simulink model "quatercar_simulinkmodel"  (R2025a)
settings: Solver=VariableStepAuto  StartTime=0.0  StopTime=10  RelTol=1e-3
values from neighbouring files (symbols this model uses):
  b = 300    [param_quatercarmodel.m]
  c = 10000    [param_quatercarmodel.m]
  c_us = 1000    [param_quatercarmodel.m]
  G = 10000    [param_quatercarmodel.m]
  m = 300    [param_quatercarmodel.m]
  m_us = 40    [param_quatercarmodel.m]
libraries: slpidlib x2
settings Model: Creator=TARUN NAIDU  LastModifiedBy=TARUN NAIDU

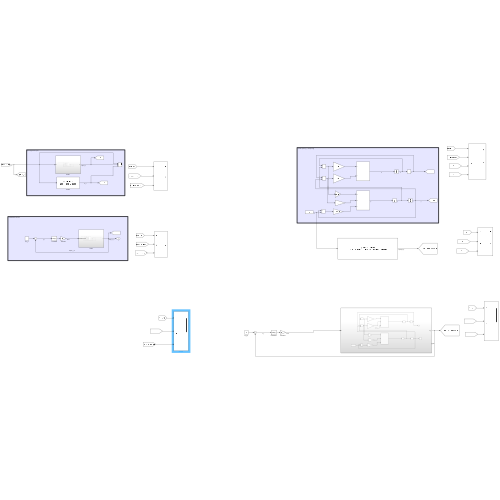
[thumbnail: Simulink's stored preview of the top-level diagram]
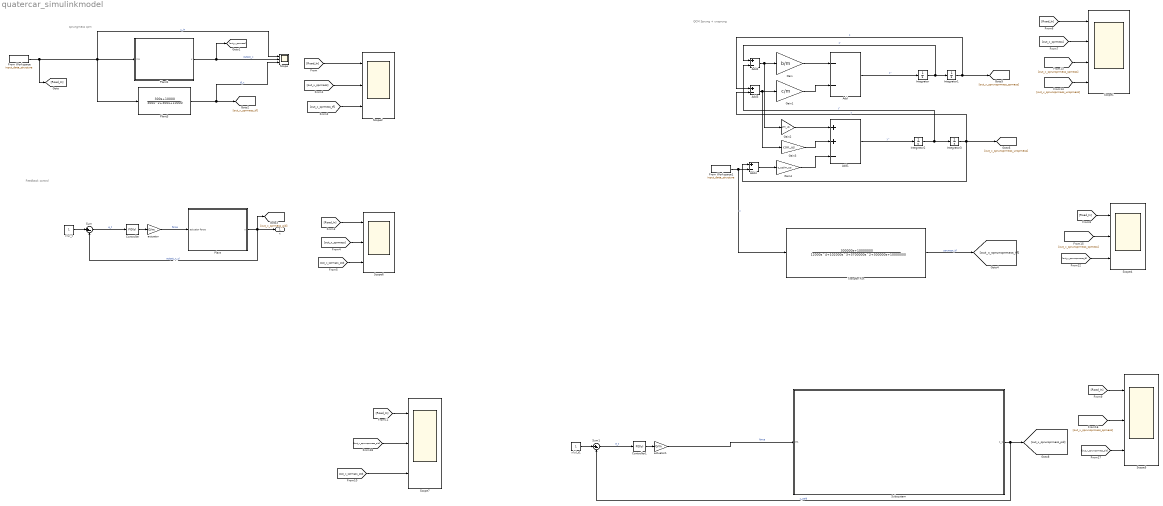
== system quatercar_simulinkmodel ==
  note: sprungmass qcm
  note: Feedback control
  note: QCM Sprung + unsprung
  Add : Sum  Inputs=--
  Add1 : Sum  Inputs=++-
  Add2 : Sum  Inputs=+-
  Add3 : Sum  Inputs=+-
  Add4 : Sum  Inputs=+-
  Controller : slpidlib/PID Controller  Controller=PID  Form=Parallel  TimeDomain=Continuous-time  UseExternalTs=off  SampleTime=-1  IntegratorMethod=Forward Euler  FilterMethod=Forward Euler  ControllerParametersSource=internal  P=4.4259  I=11.6475  UseKiTs=off  D=0.37311  UseExternalDerivativeSource=off  N=100  UseFilter=on  TunerSelectOption=Transfer Function Based (PID Tuner App)  InitialConditionSource=internal  InitialConditionForIntegrator=0  InitialConditionForFilter=0  DifferentiatorICPrevScaledInput=0  ExternalReset=none  TrackingMode=off  Kt=1  LimitOutput=off  SatLimitsSource=internal  UpperSaturationLimit=inf  LowerSaturationLimit=-inf  LinearizeAsGain=on  AntiWindupMode=none  Kb=1  LimitIntegrator=off  UpperIntegratorSaturationLimit=inf  LowerIntegratorSaturationLimit=-inf  POutMin=[]  POutMax=[]  IOutMin=[]  IOutMax=[]  DOutMin=[]  DOutMax=[]  NOutMin=[]  NOutMax=[]  SumOutMin=[]  SumOutMax=[]  SaturationOutMin=[]  SaturationOutMax=[]  PParamMin=[]  PParamMax=[]  IParamMin=[]  IParamMax=[]  DParamMin=[]  DParamMax=[]  NParamMin=[]  NParamMax=[]  KbParamMin=[]  KbParamMax=[]  KtParamMin=[]  KtParamMax=[]  KbOutMin=[]  KbOutMax=[]  KtOutMin=[]  KtOutMax=[]  IntegratorOutMin=[]  IntegratorOutMax=[]  FilterOutMin=[]  FilterOutMax=[]  SumI1OutMin=[]  SumI1OutMax=[]  SumI2OutMin=[]  SumI2OutMax=[]  SumI3OutMin=[]  SumI3OutMax=[]  SumI4OutMin=[]  SumI4OutMax=[]  SumDOutMin=[]  SumDOutMax=[]  DifferentiatorOutMin=[]  DifferentiatorOutMax=[]  FilterDiffOutCoefMin=[]  FilterDiffOutCoefMax=[]  ReciprocalOutMin=[]  ReciprocalOutMax=[]  SumDenOutMin=[]  SumDenOutMax=[]  SumNumOutMin=[]  SumNumOutMax=[]  DivideOutMin=[]  DivideOutMax=[]  UdiffTsProdOutMin=[]  UdiffTsProdOutMax=[]  NTsProdOutMin=[]  NTsProdOutMax=[]  UintegralTsProdOutMin=[]  UintegralTsProdOutMax=[]  UngainTsProdOutMin=[]  UngainTsProdOutMax=[]  ClampingZeroOutDataTypeStr=Inherit: Inherit via back propagation  ClampingZeroOutMin=[]  ClampingZeroOutMax=[]  FilterDenConstantOutDataTypeStr=Inherit: Inherit via back propagation  FilterDenConstantOutMin=[]  FilterDenConstantOutMax=[]  PCopyOutDataTypeStr=Inherit: Inherit via back propagation  PCopyOutMin=[]  PCopyOutMax=[]  NCopyOutDataTypeStr=Inherit: Inherit via back propagation  NCopyOutMin=[]  NCopyOutMax=[]  IntegratorContinuousStateAttributes=''  IntegratorStateMustResolveToSignalObject=off  IntegratorRTWStateStorageClass=Auto  FilterContinuousStateAttributes=''  FilterStateMustResolveToSignalObject=off  FilterRTWStateStorageClass=Auto  ParallelPVariant=InternalParameters  IdealPVariant=Disabled  IVariant=InternalParameters  DVariant=InternalParameters  IntegratorVariant=Continuous  SatVariant=Disabled  AWVariant=Passthrough  PCopyVariant=Disabled  TRVariant=Disabled  FdbkBlocksVariant=Forward  IdealPFdbkVariant=Disabled  SatFdbkVariant=Disabled  DerivativeFilterVariant=ContFilter  NVariant=InternalParameters  NCopyVariant=Disabled  FilterICVariant=InternalICsFilter  IntegratorICVariant=InternalICs  ExternalResetVariant=Disabled  TRSumVariant=Passthrough  SumFdbkVariant=Disabled  SumVariant=Sum_PID  TsampFilterVariant=InternalTs  TsampNgainVariant=Passthrough  TsampIntegralVariant=Disabled_SignalSpec  ExternalSaturationOutDataTypeStr=Inherit: Same as second input  DerivativeSourceVariant=ErrorSignal  PreIntVariant=InternalPreInt
  Controller1 : slpidlib/PID Controller  Controller=PID  Form=Parallel  TimeDomain=Continuous-time  UseExternalTs=off  SampleTime=-1  IntegratorMethod=Forward Euler  FilterMethod=Forward Euler  ControllerParametersSource=internal  P=4.8162  I=3.2747  UseKiTs=off  D=1.5851  UseExternalDerivativeSource=off  N=100  UseFilter=on  TunerSelectOption=Transfer Function Based (PID Tuner App)  InitialConditionSource=internal  InitialConditionForIntegrator=0  InitialConditionForFilter=0  DifferentiatorICPrevScaledInput=0  ExternalReset=none  TrackingMode=off  Kt=1  LimitOutput=off  SatLimitsSource=internal  UpperSaturationLimit=inf  LowerSaturationLimit=-inf  LinearizeAsGain=on  AntiWindupMode=none  Kb=1  LimitIntegrator=off  UpperIntegratorSaturationLimit=inf  LowerIntegratorSaturationLimit=-inf  POutMin=[]  POutMax=[]  IOutMin=[]  IOutMax=[]  DOutMin=[]  DOutMax=[]  NOutMin=[]  NOutMax=[]  SumOutMin=[]  SumOutMax=[]  SaturationOutMin=[]  SaturationOutMax=[]  PParamMin=[]  PParamMax=[]  IParamMin=[]  IParamMax=[]  DParamMin=[]  DParamMax=[]  NParamMin=[]  NParamMax=[]  KbParamMin=[]  KbParamMax=[]  KtParamMin=[]  KtParamMax=[]  KbOutMin=[]  KbOutMax=[]  KtOutMin=[]  KtOutMax=[]  IntegratorOutMin=[]  IntegratorOutMax=[]  FilterOutMin=[]  FilterOutMax=[]  SumI1OutMin=[]  SumI1OutMax=[]  SumI2OutMin=[]  SumI2OutMax=[]  SumI3OutMin=[]  SumI3OutMax=[]  SumI4OutMin=[]  SumI4OutMax=[]  SumDOutMin=[]  SumDOutMax=[]  DifferentiatorOutMin=[]  DifferentiatorOutMax=[]  FilterDiffOutCoefMin=[]  FilterDiffOutCoefMax=[]  ReciprocalOutMin=[]  ReciprocalOutMax=[]  SumDenOutMin=[]  SumDenOutMax=[]  SumNumOutMin=[]  SumNumOutMax=[]  DivideOutMin=[]  DivideOutMax=[]  UdiffTsProdOutMin=[]  UdiffTsProdOutMax=[]  NTsProdOutMin=[]  NTsProdOutMax=[]  UintegralTsProdOutMin=[]  UintegralTsProdOutMax=[]  UngainTsProdOutMin=[]  UngainTsProdOutMax=[]  ClampingZeroOutDataTypeStr=Inherit: Inherit via back propagation  ClampingZeroOutMin=[]  ClampingZeroOutMax=[]  FilterDenConstantOutDataTypeStr=Inherit: Inherit via back propagation  FilterDenConstantOutMin=[]  FilterDenConstantOutMax=[]  PCopyOutDataTypeStr=Inherit: Inherit via back propagation  PCopyOutMin=[]  PCopyOutMax=[]  NCopyOutDataTypeStr=Inherit: Inherit via back propagation  NCopyOutMin=[]  NCopyOutMax=[]  IntegratorContinuousStateAttributes=''  IntegratorStateMustResolveToSignalObject=off  IntegratorRTWStateStorageClass=Auto  FilterContinuousStateAttributes=''  FilterStateMustResolveToSignalObject=off  FilterRTWStateStorageClass=Auto  ParallelPVariant=InternalParameters  IdealPVariant=Disabled  IVariant=InternalParameters  DVariant=InternalParameters  IntegratorVariant=Continuous  SatVariant=Disabled  AWVariant=Passthrough  PCopyVariant=Disabled  TRVariant=Disabled  FdbkBlocksVariant=Forward  IdealPFdbkVariant=Disabled  SatFdbkVariant=Disabled  DerivativeFilterVariant=ContFilter  NVariant=InternalParameters  NCopyVariant=Disabled  FilterICVariant=InternalICsFilter  IntegratorICVariant=InternalICs  ExternalResetVariant=Disabled  TRSumVariant=Passthrough  SumFdbkVariant=Disabled  SumVariant=Sum_PID  TsampFilterVariant=InternalTs  TsampNgainVariant=Passthrough  TsampIntegralVariant=Disabled_SignalSpec  ExternalSaturationOutDataTypeStr=Inherit: Same as second input  DerivativeSourceVariant=ErrorSignal  PreIntVariant=InternalPreInt
  From Workspace : FromWorkspace  VariableName=input_data_structure
  From Workspace1 : FromWorkspace  VariableName=input_data_structure
  Gain : Gain  Gain=b/m
  Gain1 : Gain  Gain=c/m
  Gain2 : Gain  Gain=b/m_us
  Gain3 : Gain  Gain=c/m_us
  Gain4 : Gain  Gain=c_us/m_us
  Integrator{,1..3} (4 alike) : Integrator
  Plant : Subsystem
  Plant1 : Subsystem
  Plant3 : TransferFcn  Numerator=[300, 10000]  Denominator=[300 300 10000]
  Scope{,2,4..7} (6 alike) : Scope  NumInputPorts=3
      Scope settings: ActiveDisplayYMinimum=-9.7561874172435648  ActiveDisplayYMaximum=3.57864772968778
      Scope2 settings: ActiveDisplayYMinimum=-8.5975098735080913  ActiveDisplayYMaximum=6.5080880547958344  DataLoggingVariableName=ScopeData2
      Scope4 settings: ActiveDisplayYMinimum=-3.0149645967073719  ActiveDisplayYMaximum=2.3447311686554464  DataLoggingVariableName=ScopeData4
      Scope5 settings: ActiveDisplayYMinimum=-3.280617062263274  ActiveDisplayYMaximum=2.7105701768573249  DataLoggingVariableName=ScopeData6
      Scope6 settings: ActiveDisplayYMinimum=-8.3191474885252319  ActiveDisplayYMaximum=6.0700672911799529  DataLoggingVariableName=ScopeData7
      Scope7 settings: ActiveDisplayYMinimum=-3.280617062263274  ActiveDisplayYMaximum=2.7105701768573249  DataLoggingVariableName=ScopeData8
  Scope1 : Scope  NumInputPorts=4
      settings: ActiveDisplayYMinimum=-5.8988564281329783  ActiveDisplayYMaximum=6.7403880590338119
  Subsystem : Subsystem
  Sum : Sum  Inputs=|+-
  Sum1 : Sum  Inputs=|+-
  Transfer Fcn : TransferFcn  Numerator=[300000 10000000]  Denominator=[12000 102000 3700000 300000 10000000]
  actuator : Gain  Gain=G/m
  actuator1 : Gain  Gain=G/m
  x(u)_t : Constant
  x(u)_t1 : Constant
  x : Outport
  wires:
  x(u)_t/1 -> Sum/1
  Sum/1 -> Controller/1  "e_t"
  Controller/1 -> actuator/1
  Plant/1(x) -> [out_x_sprmass_pid], Sum/2, x/1  "output_x_cl"
  actuator/1 -> Plant/1(actuator force)  "force"
  Plant1/1(x) -> [out_x_sprmass], Scope/2  "output_x"
  From Workspace/1 -> Plant3/1, Scope/1, Plant1/1(In1), [Road_In]  "z_in"
  Plant3/1 -> Scope/3, [out_x_sprmass_tf]  "tf_x"
  [Road_In] -> Scope2/1
  [out_x_sprmass] -> Scope2/2
  [out_x_sprmass_tf] -> Scope2/3
  [Road_In] -> Scope6/1
  [out_x_sprmass] -> Scope6/2
  [out_x_sprmass_pid] -> Scope6/3
  [Road_In] -> Scope4/1
  [Road_In] -> Scope5/1
  Transfer Fcn/1 -> [out_x_sprunsprmass_tf]  "sprunspr_tf"
  Gain1/1 -> Add/2
  Sum1/1 -> Controller1/1  "e_t"
  From Workspace1/1 -> Transfer Fcn/1, Add4/2  "z"
  Integrator/1 -> Add2/1, Integrator1/1  "z'"
  Gain/1 -> Add/1
  Integrator2/1 -> Add2/2, Integrator3/1  "y'"
  Subsystem/1(z_s) -> [out_x_sprunsprmass_pid], Sum1/2  "z_spid"
  Gain4/1 -> Add1/3
  [out_x_sprmass] -> Scope1/2
  Add2/1 -> Gain2/1, Gain/1
  [Road_In] -> Scope1/1
  Integrator3/1 -> [out_x_sprunsprmass_unspmass], Add4/1, Add3/2  "y"
  Gain2/1 -> Add1/1
  Gain3/1 -> Add1/2
  Add1/1 -> Integrator2/1  "y''"
  Controller1/1 -> actuator1/1
  x(u)_t1/1 -> Sum1/1
  Add4/1 -> Gain4/1
  Integrator1/1 -> Add3/1, [out_x_sprunsprmass_spmass]  "z"
  actuator1/1 -> Subsystem/1(In1)  "force"
  Add3/1 -> Gain3/1, Gain1/1
  Add/1 -> Integrator/1  "z''"
  [Road_In] -> Scope7/1
  [out_x_sprunsprmass_tf] -> Scope4/3
  [out_x_sprunsprmass_spmass] -> Scope1/3
  [out_x_sprunsprmass_unspmass] -> Scope1/4
  [out_x_sprunsprmass_spmass] -> Scope4/2
  [out_x_sprmass_pid] -> Scope7/3
  [out_x_sprunsprmass_spmass] -> Scope5/2
  [out_x_sprunsprmass_pid] -> Scope5/3
  [out_x_sprunsprmass_pid] -> Scope7/2

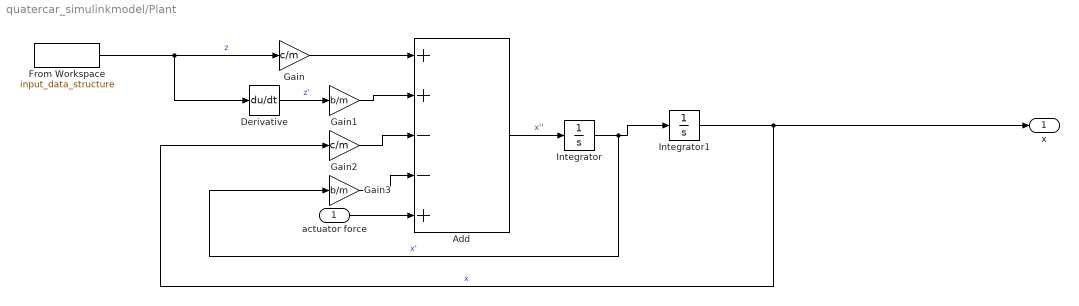
== system quatercar_simulinkmodel/Plant ==
  actuator force : Inport
  Add : Sum  Inputs=++--+
  Derivative : Derivative
  From Workspace : FromWorkspace  VariableName=input_data_structure
  Gain : Gain  Gain=c/m
  Gain1 : Gain  Gain=b/m
  Gain2 : Gain  Gain=c/m
  Gain3 : Gain  Gain=b/m
  Integrator : Integrator  InitialCondition=0.12
  Integrator1 : Integrator  InitialCondition=0.2
  x : Outport
  wires:
  Integrator/1 -> Gain3/1, Integrator1/1  "x'"
  Add/1 -> Integrator/1  "x''"
  Integrator1/1 -> x/1, Gain2/1  "x"
  From Workspace/1 -> Derivative/1, Gain/1  "z"
  Gain/1 -> Add/1
  Gain1/1 -> Add/2
  Derivative/1 -> Gain1/1  "z'"
  Gain3/1 -> Add/4
  Gain2/1 -> Add/3
  actuator force/1 -> Add/5

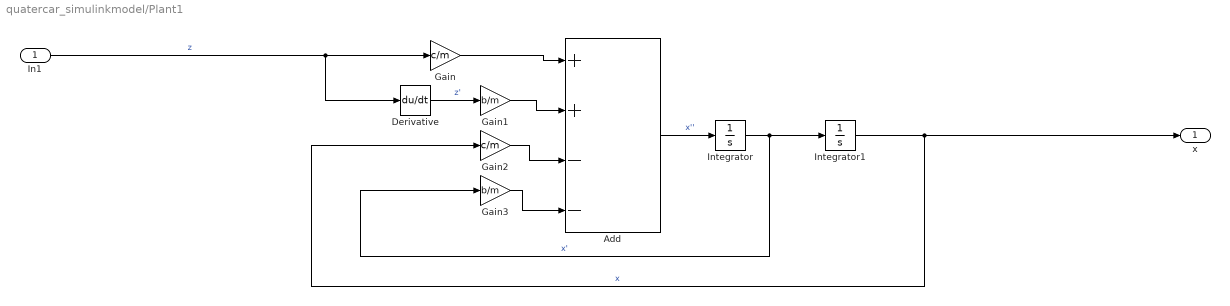
== system quatercar_simulinkmodel/Plant1 ==
  In1 : Inport
  Add : Sum  Inputs=++--
  Derivative : Derivative
  Gain : Gain  Gain=c/m
  Gain1 : Gain  Gain=b/m
  Gain2 : Gain  Gain=c/m
  Gain3 : Gain  Gain=b/m
  Integrator : Integrator  InitialCondition=0.12
  Integrator1 : Integrator  InitialCondition=0.2
  x : Outport
  wires:
  Integrator/1 -> Gain3/1, Integrator1/1  "x'"
  Add/1 -> Integrator/1  "x''"
  Integrator1/1 -> x/1, Gain2/1  "x"
  In1/1 -> Derivative/1, Gain/1  "z"
  Gain/1 -> Add/1
  Gain1/1 -> Add/2
  Derivative/1 -> Gain1/1  "z'"
  Gain3/1 -> Add/4
  Gain2/1 -> Add/3

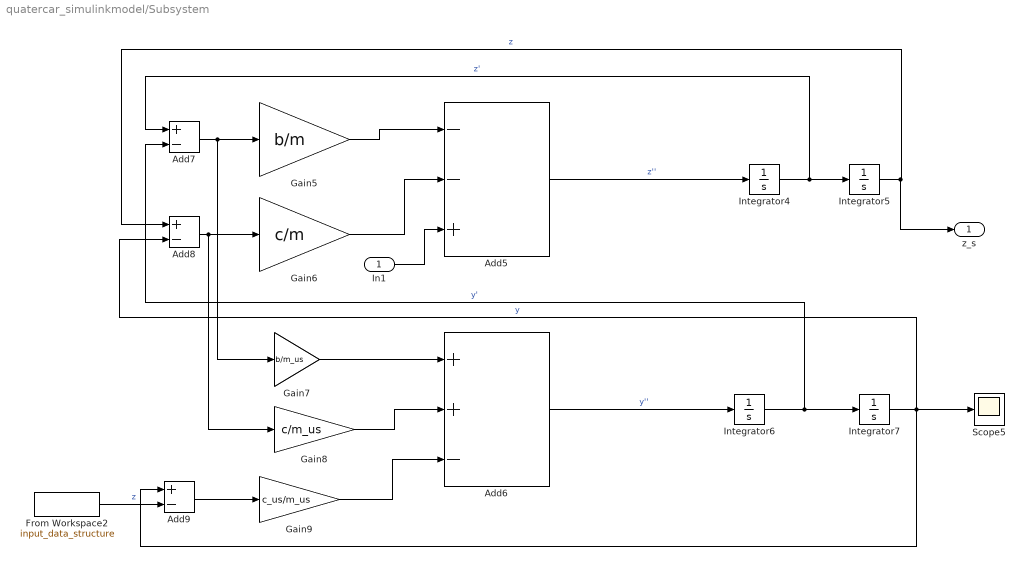
== system quatercar_simulinkmodel/Subsystem ==
  In1 : Inport
  Add5 : Sum  Inputs=--+
  Add6 : Sum  Inputs=++-
  Add7 : Sum  Inputs=+-
  Add8 : Sum  Inputs=+-
  Add9 : Sum  Inputs=+-
  From Workspace2 : FromWorkspace  VariableName=input_data_structure
  Gain5 : Gain  Gain=b/m
  Gain6 : Gain  Gain=c/m
  Gain7 : Gain  Gain=b/m_us
  Gain8 : Gain  Gain=c/m_us
  Gain9 : Gain  Gain=c_us/m_us
  Integrator{4..7} (4 alike) : Integrator
  Scope5 : Scope
      settings: DataLoggingVariableName=ScopeData5
  z_s : Outport
  wires:
  Add8/1 -> Gain8/1, Gain6/1
  Integrator6/1 -> Add7/2, Integrator7/1  "y'"
  Integrator5/1 -> z_s/1, Add8/1  "z"
  From Workspace2/1 -> Add9/2  "z"
  Integrator7/1 -> Add9/1, Add8/2, Scope5/1  "y"
  Add5/1 -> Integrator4/1  "z''"
  Add6/1 -> Integrator6/1  "y''"
  Gain8/1 -> Add6/2
  Gain6/1 -> Add5/2
  Gain7/1 -> Add6/1
  Integrator4/1 -> Add7/1, Integrator5/1  "z'"
  Add9/1 -> Gain9/1
  Gain9/1 -> Add6/3
  Add7/1 -> Gain7/1, Gain5/1
  Gain5/1 -> Add5/1
  In1/1 -> Add5/3
